simulink model "hw2sim2"  (R2024b)
settings: Solver=FixedStepAuto  StartTime=0.0  StopTime=5  FixedStep=1/86400  RelTol=1e-3
settings Model: Creator=yugpn  LastModifiedBy=JTerr

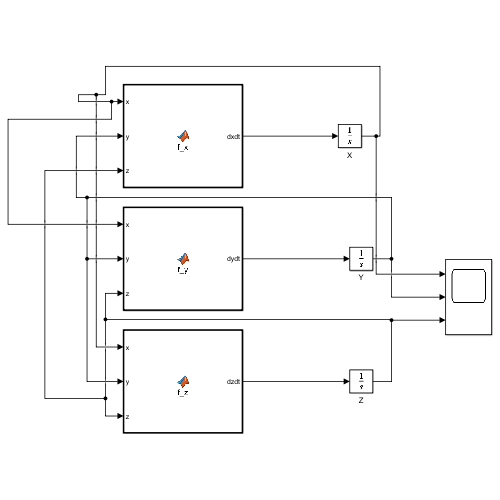
[thumbnail: Simulink's stored preview of the top-level diagram]
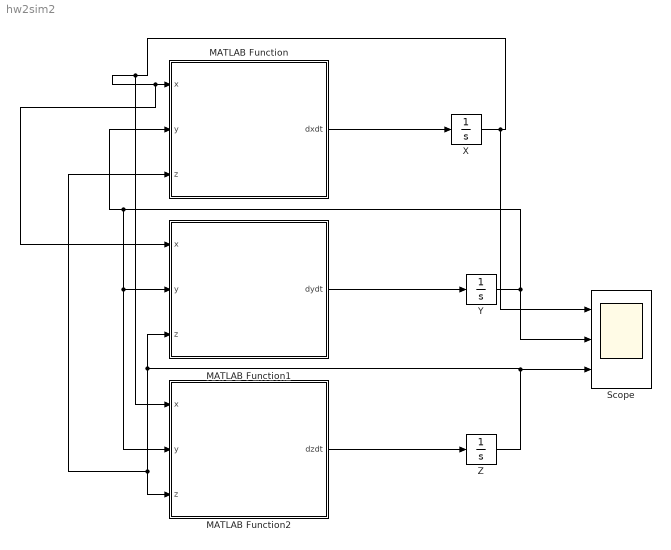
== system hw2sim2 ==
  MATLAB Function : MATLAB Function  TreatAsAtomicUnit=on
  MATLAB Function1 : MATLAB Function  TreatAsAtomicUnit=on
  MATLAB Function2 : MATLAB Function  TreatAsAtomicUnit=on
  Scope : Scope  NumInputPorts=3
  X : Integrator
  Y : Integrator
  Z : Integrator
  wires:
  MATLAB Function2/1(dzdt) -> Z/1
  MATLAB Function1/1(dydt) -> Y/1
  MATLAB Function/1(dxdt) -> X/1
  X/1 -> Scope/1, MATLAB Function2/1(x), MATLAB Function1/1(x), MATLAB Function/1(x)
  Y/1 -> MATLAB Function/2(y), MATLAB Function2/2(y), MATLAB Function1/2(y), Scope/2
  Z/1 -> Scope/3, MATLAB Function1/3(z), MATLAB Function2/3(z), MATLAB Function/3(z)

== matlab function hw2sim2/MATLAB Function ==
  data: x input; dxdt output; y input; z input
function dxdt = f_x(x, y, z)
    kx = 2;
    x0e = 10;
    alpha = 10;
    beta = 2;
    k1 = alpha - beta * z;
    dxdt = kx * (x0e - x) - k1 * x * y;
end

== matlab function hw2sim2/MATLAB Function2 ==
  data: x input; dzdt output; y input; z input
function dzdt = f_z(x, y, z)
    alpha = 10;
    beta = 2;
    gamma = 2;
    k1 = alpha - beta * z;
    dzdt = k1 * x * y - gamma * z;
end

== matlab function hw2sim2/MATLAB Function1 ==
  data: x input; dydt output; y input; z input
function dydt = f_y(x, y, z)
    ky = 3;
    y0e = 6;
    alpha = 10;
    beta = 2;
    k1 = alpha - beta * z;
    dydt = ky * (y0e - y) - k1 * x * y;
end
